simulink model "URM"  (R2023b)
settings: Solver=VariableStepAuto  StartTime=0.0  StopTime=10.0  RelTol=1e-3
undefined symbols (not defined in the file): kd, ki, kp
settings Model: Creator=tomasz  LastModifiedBy=tomasz

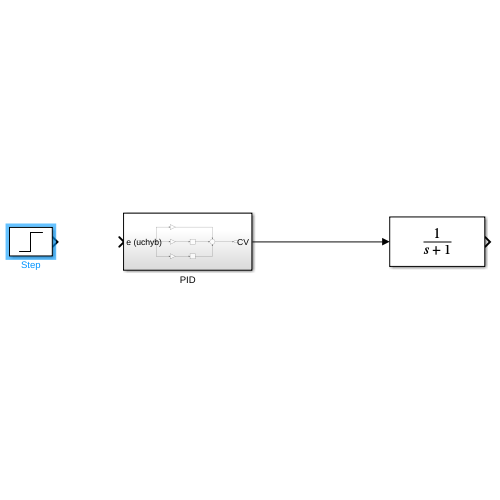
[thumbnail: Simulink's stored preview of the top-level diagram]
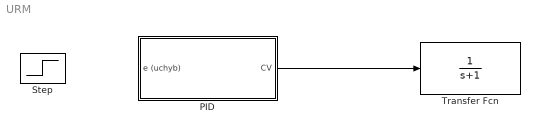
== system URM ==
  PID : Subsystem
  Step : Step  SampleTime=0
  Transfer Fcn : TransferFcn  Denominator=[1 1]
  wires:
  PID/1(CV) -> Transfer Fcn/1

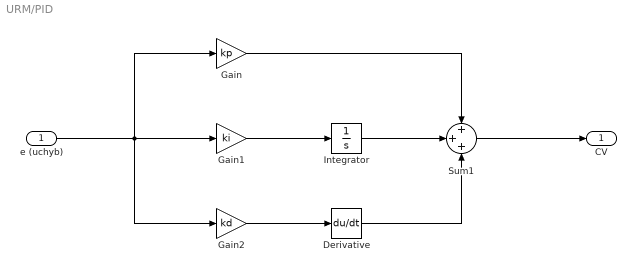
== system URM/PID ==
  e (uchyb) : Inport
  Derivative : Derivative
  Gain : Gain  Gain=kp
  Gain1 : Gain  Gain=ki
  Gain2 : Gain  Gain=kd
  Integrator : Integrator
  Sum1 : Sum  Inputs=+++
  CV : Outport
  wires:
  Derivative/1 -> Sum1/3
  Gain1/1 -> Integrator/1
  Gain2/1 -> Derivative/1
  Integrator/1 -> Sum1/2
  e (uchyb)/1 -> Gain1/1, Gain/1, Gain2/1
  Gain/1 -> Sum1/1
  Sum1/1 -> CV/1
